simulink library "debug_tools"  (Simulink 7.4)
settings: Solver=ode45  StartTime=0.0  StopTime=10.0  RelTol=1e-3
libraries: xbsIndex_r4 x6, casper_library_misc x2
settings Model: Creator=mwagner  LastModifiedBy=mwagner

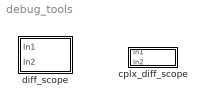
== system debug_tools ==
  cplx_diff_scope : Subsystem  mask{input_bit_width=0, input_bin_pt=0}
  diff_scope : Subsystem

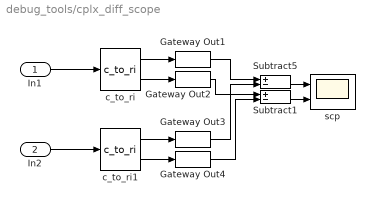
== system debug_tools/cplx_diff_scope ==
  In1 : Inport
  In2 : Inport  Port=2
  Gateway Out{1..4} (4 alike) : xbsIndex_r4/Gateway Out  hdl_port=on  timing_constraint=None  locs_specified=off  LOCs={}  block_type=gatewayout
      settings: infoedit="Gateway out block.  Converts Xilinx fixed point inputs into ouputs of type Simulink integer, double, or fixed point.<br><br>Hardware notes:  In hardware these blocks become top level output ports or are discarded, depending on how they are configured."  block_version=11.4
  Subtract1 : Sum  Inputs=+-  OutDataType=fixdt(1, 16)  OutScaling=2^-10
  Subtract5 : Sum  Inputs=+-  OutDataType=fixdt(1, 16)  OutScaling=2^-10
  c_to_ri : casper_library_misc/c_to_ri  SystemSampleTime=-1  n_bits=input_bit_width  bin_pt=input_bin_pt
      settings: AttributesFormatString=0_0 r/i
  c_to_ri1 : casper_library_misc/c_to_ri  SystemSampleTime=-1  n_bits=input_bit_width  bin_pt=input_bin_pt
      settings: AttributesFormatString=0_0 r/i
  scp : Scope  NumInputPorts=2
      settings: YMin=-5~-5  YMax=5~5  SaveName=ScopeData3
  wires:
  Subtract5/1 -> scp/1
  In1/1 -> c_to_ri/1
  In2/1 -> c_to_ri1/1
  c_to_ri/1 -> Gateway Out1/1
  c_to_ri/2 -> Gateway Out2/1
  c_to_ri1/1 -> Gateway Out3/1
  c_to_ri1/2 -> Gateway Out4/1
  Subtract1/1 -> scp/2
  Gateway Out1/1 -> Subtract5/1
  Gateway Out2/1 -> Subtract1/1
  Gateway Out3/1 -> Subtract5/2
  Gateway Out4/1 -> Subtract1/2

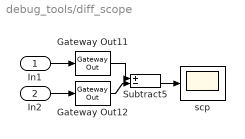
== system debug_tools/diff_scope ==
  In1 : Inport
  In2 : Inport  Port=2
  Gateway Out11 : xbsIndex_r4/Gateway Out  hdl_port=on  timing_constraint=None  locs_specified=off  LOCs={}  block_type=gatewayout
      settings: infoedit="Gateway out block.  Converts Xilinx fixed point inputs into ouputs of type Simulink integer, double, or fixed point.<br><br>Hardware notes:  In hardware these blocks become top level output ports or are discarded, depending on how they are configured."  block_version=11.4
  Gateway Out12 : xbsIndex_r4/Gateway Out  hdl_port=on  timing_constraint=None  locs_specified=off  LOCs={}  block_type=gatewayout
      settings: infoedit="Gateway out block.  Converts Xilinx fixed point inputs into ouputs of type Simulink integer, double, or fixed point.<br><br>Hardware notes:  In hardware these blocks become top level output ports or are discarded, depending on how they are configured."  block_version=11.4
  Subtract5 : Sum  Inputs=+-  OutDataType=fixdt(1, 16)  OutScaling=2^-10
  scp : Scope
      settings: SaveName=ScopeData3
  wires:
  Subtract5/1 -> scp/1
  Gateway Out11/1 -> Subtract5/1
  Gateway Out12/1 -> Subtract5/2
  In1/1 -> Gateway Out11/1
  In2/1 -> Gateway Out12/1
